simulink model "untitled"  (R2014b)
settings: Solver=ode45  StartTime=0.0  StopTime=10.0  RelTol=1e-3
settings Model: Creator=maksimka  LastModifiedBy=maksimka

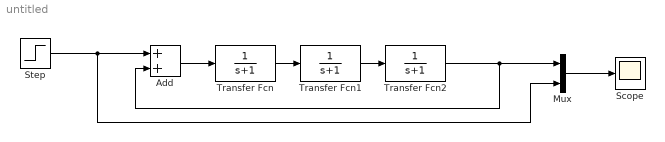
== system untitled ==
  Add : Sum
  Mux : Mux  Inputs=2
  Scope : Scope
  Step : Step  SampleTime=0
  Transfer Fcn : TransferFcn  Denominator=[1 1]
  Transfer Fcn1 : TransferFcn  Denominator=[1 1]
  Transfer Fcn2 : TransferFcn  Denominator=[1 1]
  wires:
  Transfer Fcn/1 -> Transfer Fcn1/1
  Step/1 -> Mux/2, Add/1
  Transfer Fcn1/1 -> Transfer Fcn2/1
  Transfer Fcn2/1 -> Add/2, Mux/1
  Mux/1 -> Scope/1
  Add/1 -> Transfer Fcn/1
